simulink model "Pacejka_Lateral_Tyre_Model"  (R2024a)
settings: Solver=VariableStepAuto  StartTime=0.0  StopTime=10.0  RelTol=1e-3
values from neighbouring files (symbols this model uses):
  a1 = -1e-5    (= -1e-05)    [Longitudinal_Braking_Parameters.m]    (also in Pacejka_lateral_parameters.m)
  a2 = 1.25    [Longitudinal_Braking_Parameters.m]    (also in Pacejka_lateral_parameters.m)
  B = 4.1576    [Longitudinal_Braking_Parameters.m]    (also in Pacejka_lateral_parameters.m = 0.1453)
  C = 1.7810    (= 1.781)    [Longitudinal_Braking_Parameters.m]    (also in Pacejka_lateral_parameters.m = 1.5511)
settings Model: Creator=gaurimorjaria  LastModifiedBy=gaurimorjaria

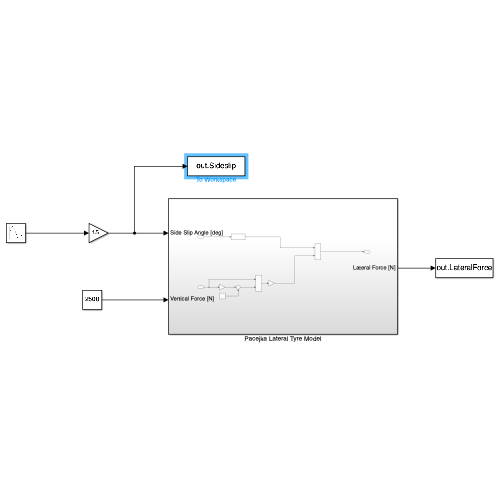
[thumbnail: Simulink's stored preview of the top-level diagram]
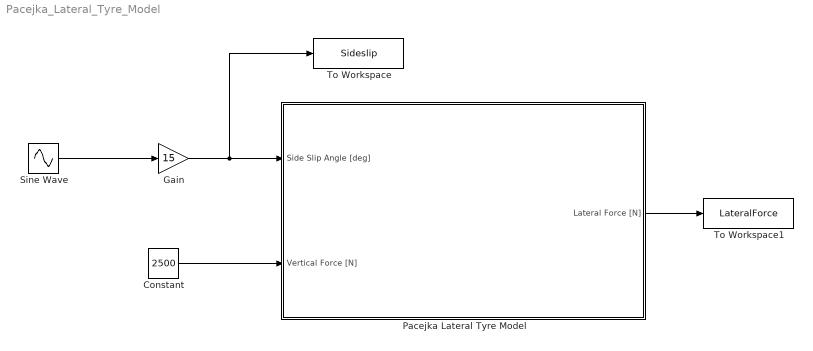
== system Pacejka_Lateral_Tyre_Model ==
  Constant : Constant  Value=2500
  Gain : Gain  Gain=15
  Pacejka Lateral Tyre Model : Subsystem
  Sine Wave : Sin  SampleTime=0
  To Workspace : ToWorkspace  VariableName=Sideslip  SaveFormat=Timeseries  SampleTime=-1
      settings: Save2DSignal=2-D array (concatenate along first dimension)
  To Workspace1 : ToWorkspace  VariableName=LateralForce  SaveFormat=Timeseries  SampleTime=-1
      settings: Save2DSignal=2-D array (concatenate along first dimension)
  wires:
  Constant/1 -> Pacejka Lateral Tyre Model/2(Vertical Force [N])
  Sine Wave/1 -> Gain/1
  Gain/1 -> To Workspace/1, Pacejka Lateral Tyre Model/1(Side Slip Angle [deg])
  Pacejka Lateral Tyre Model/1(Lateral Force [N]) -> To Workspace1/1

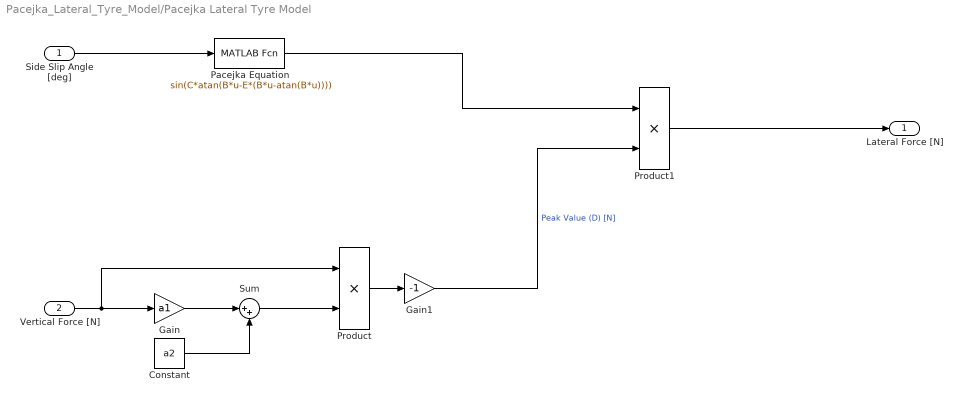
== system Pacejka_Lateral_Tyre_Model/Pacejka Lateral Tyre Model ==
  Side Slip Angle [deg] : Inport
  Vertical Force [N] : Inport  Port=2
  Constant : Constant  Value=a2
  Gain : Gain  Gain=a1
  Gain1 : Gain  Gain=-1
  Pacejka Equation : MATLABFcn  MATLABFcn=sin(C*atan(B*u-E*(B*u-atan(B*u))))
  Product : Product
  Product1 : Product
  Sum : Sum  Inputs=|++
  Lateral Force [N] : Outport
  wires:
  Vertical Force [N]/1 -> Product/1, Gain/1
  Gain/1 -> Sum/1
  Constant/1 -> Sum/2
  Sum/1 -> Product/2
  Product/1 -> Gain1/1
  Gain1/1 -> Product1/2  "Peak Value (D) [N]"
  Product1/1 -> Lateral Force [N]/1
  Side Slip Angle [deg]/1 -> Pacejka Equation/1
  Pacejka Equation/1 -> Product1/1
